simulink library "DAMA_lib"  (Simulink 6.6)
undefined symbols (not defined in the file or in its folder): aa2rot, D, DiscIntNeverNeededParam, DRprogressbar, epsilon, Kd, Ko, Kp, manip, manipulator, path_des, Q, q0, q_d0, rho, robot, show_3D, StartTime, subs, Ts, VR_handle, vrmfunc
libraries: DAMA_lib x7, vrlib x1, simulink x1
(part 4 of 4)

== system DAMA_lib/Kinematics/Transpose Jacobian Inverse Kinematics/Subsystem/cross product1 ==
  u : Inport
  v : Inport  Port=2
  Mux1 : Mux  Inputs=2
  cross : MATLABFcn  MATLABFcn=cross(u(1:3),u(4:6))  Output1D=off
  u x v : Outport
  wires:
  v/1 -> Mux1/2
  cross/1 -> u x v/1
  u/1 -> Mux1/1
  Mux1/1 -> cross/1

== system DAMA_lib/Kinematics/Transpose Jacobian Inverse Kinematics/Subsystem/cross product2 ==
  u : Inport
  v : Inport  Port=2
  Mux1 : Mux  Inputs=2
  cross : MATLABFcn  MATLABFcn=cross(u(1:3),u(4:6))  Output1D=off
  u x v : Outport
  wires:
  Mux1/1 -> cross/1
  u/1 -> Mux1/1
  cross/1 -> u x v/1
  v/1 -> Mux1/2

== system DAMA_lib/Kinematics/Transpose Jacobian Inverse Kinematics/Subsystem/cross product3 ==
  u : Inport
  v : Inport  Port=2
  Mux1 : Mux  Inputs=2
  cross : MATLABFcn  MATLABFcn=cross(u(1:3),u(4:6))  Output1D=off
  u x v : Outport
  wires:
  v/1 -> Mux1/2
  cross/1 -> u x v/1
  u/1 -> Mux1/1
  Mux1/1 -> cross/1
